simulink model "Marine_LocoMotive_UAV_est_git"  (R2018a)
settings: Solver=ode4  StartTime=0.0  StopTime=40  FixedStep=T  MaxStep=2*T  MinStep=T  RelTol=1e-4
values from neighbouring files (symbols this model uses):
  a_11 = 0.05*m_b    (= 0.625)    [Marine_LocoMotive_UAV_est_git_parameters.m]    (also in Marine_LocoMotive_UAV_medium_est_git_parameters.m = 1.6875; heave_dynamics_chart.m)
  a_33 = m_b    (= 12.5)    [Marine_LocoMotive_UAV_est_git_parameters.m]    (also in Marine_LocoMotive_UAV_medium_est_git_parameters.m = 33.75; heave_dynamics_chart.m)
  A_w = 1*3.3/2    (= 1.65)    [Marine_LocoMotive_UAV_est_git_parameters.m]    (also in Marine_LocoMotive_UAV_medium_est_git_parameters.m = 0.6)
  A_w2 = 1*1.2/2    (= 0.6)    [Marine_LocoMotive_UAV_est_git_parameters.m]    (also in Marine_LocoMotive_UAV_medium_est_git_parameters.m = 0.305)
  Ac = 0.0331    [Marine_LocoMotive_UAV_est_git_parameters.m]    (also in Marine_LocoMotive_UAV_medium_est_git_parameters.m = 0.422)
  alpha_bar = pi/4    (= 0.785398163397)    [Marine_LocoMotive_UAV_est_git_parameters.m]    (also in Marine_LocoMotive_UAV_medium_est_git_parameters.m; heave_dynamics_chart.m = pi/4*sign(V_bar(j)))
  Am = sysd.denominator{1}    [Marine_LocoMotive_UAV_est_git_parameters.m]    (also in Marine_LocoMotive_UAV_medium_est_git_parameters.m)
  Am1_LPF = sysd.denominator{1}    [Marine_LocoMotive_UAV_est_git_parameters.m]    (also in Marine_LocoMotive_UAV_medium_est_git_parameters.m)
  Am2_LPF = sysd.denominator{1}    [Marine_LocoMotive_UAV_est_git_parameters.m]    (also in Marine_LocoMotive_UAV_medium_est_git_parameters.m)
  Am_asw_LPF = sysd.denominator{1}    [Marine_LocoMotive_UAV_est_git_parameters.m]    (also in Marine_LocoMotive_UAV_medium_est_git_parameters.m)
  Am_coup_LPF = sysd.denominator{1}    [Marine_LocoMotive_UAV_est_git_parameters.m]    (also in Marine_LocoMotive_UAV_medium_est_git_parameters.m)
  Am_fast_coup_LPF = sysd.denominator{1}    [Marine_LocoMotive_UAV_est_git_parameters.m]    (also in Marine_LocoMotive_UAV_medium_est_git_parameters.m)
  Am_rdeL_LPF = sysd.denominator{1}    [Marine_LocoMotive_UAV_est_git_parameters.m]    (also in Marine_LocoMotive_UAV_medium_est_git_parameters.m)
  Am_reL_LPF = sysd.denominator{1}    [Marine_LocoMotive_UAV_est_git_parameters.m]    (also in Marine_LocoMotive_UAV_medium_est_git_parameters.m)
  Am_rref20_LPF = sysd.denominator{1}    [Marine_LocoMotive_UAV_est_git_parameters.m]    (also in Marine_LocoMotive_UAV_medium_est_git_parameters.m)
  Am_rref_LPF = sysd.denominator{1}    [Marine_LocoMotive_UAV_est_git_parameters.m]    (also in Marine_LocoMotive_UAV_medium_est_git_parameters.m)
  AmAlpha_LPF = sysd.denominator{1}    [Marine_LocoMotive_UAV_est_git_parameters.m]    (also in Marine_LocoMotive_UAV_medium_est_git_parameters.m)
  Amp_sf = 3    [Marine_LocoMotive_UAV_est_git_parameters.m]    (also in Marine_LocoMotive_UAV_medium_est_git_parameters.m)
  Amp_sf_rp = 0.05*m_u*g    (= 0.8829)    [Marine_LocoMotive_UAV_est_git_parameters.m]    (also in Marine_LocoMotive_UAV_medium_est_git_parameters.m = 9.56475)
  AmV_LPF = sysd.denominator{1}    [Marine_LocoMotive_UAV_est_git_parameters.m]    (also in Marine_LocoMotive_UAV_medium_est_git_parameters.m)
  AmZ_LPF = sysd.denominator{1}    [Marine_LocoMotive_UAV_est_git_parameters.m]    (also in Marine_LocoMotive_UAV_medium_est_git_parameters.m)
  b_11 = 0    [Marine_LocoMotive_UAV_est_git_parameters.m]    (also in Marine_LocoMotive_UAV_medium_est_git_parameters.m; heave_dynamics_chart.m)
  b_33 = 2*m_b*omega_h    (= 19.6349540849)    [Marine_LocoMotive_UAV_est_git_parameters.m]    (also in Marine_LocoMotive_UAV_medium_est_git_parameters.m = 84.8230016469; buoyancy_calc.m = 4.18879020479; heave_dynamics_chart.m = 2*m_b*omega_h)
  Bm = sysd.numerator{1}    [Marine_LocoMotive_UAV_est_git_parameters.m]    (also in Marine_LocoMotive_UAV_medium_est_git_parameters.m)
  Bm1_LPF = sysd.numerator{1}    [Marine_LocoMotive_UAV_est_git_parameters.m]    (also in Marine_LocoMotive_UAV_medium_est_git_parameters.m)
  Bm2_LPF = sysd.numerator{1}    [Marine_LocoMotive_UAV_est_git_parameters.m]    (also in Marine_LocoMotive_UAV_medium_est_git_parameters.m)
  Bm_asw_LPF = sysd.numerator{1}    [Marine_LocoMotive_UAV_est_git_parameters.m]    (also in Marine_LocoMotive_UAV_medium_est_git_parameters.m)
  Bm_coup_LPF = sysd.numerator{1}    [Marine_LocoMotive_UAV_est_git_parameters.m]    (also in Marine_LocoMotive_UAV_medium_est_git_parameters.m)
  Bm_fast_coup_LPF = sysd.numerator{1}    [Marine_LocoMotive_UAV_est_git_parameters.m]    (also in Marine_LocoMotive_UAV_medium_est_git_parameters.m)
  Bm_rdeL_LPF = sysd.numerator{1}    [Marine_LocoMotive_UAV_est_git_parameters.m]    (also in Marine_LocoMotive_UAV_medium_est_git_parameters.m)
  Bm_reL_LPF = sysd.numerator{1}    [Marine_LocoMotive_UAV_est_git_parameters.m]    (also in Marine_LocoMotive_UAV_medium_est_git_parameters.m)
  Bm_rref20_LPF = sysd.numerator{1}    [Marine_LocoMotive_UAV_est_git_parameters.m]    (also in Marine_LocoMotive_UAV_medium_est_git_parameters.m)
  Bm_rref_LPF = sysd.numerator{1}    [Marine_LocoMotive_UAV_est_git_parameters.m]    (also in Marine_LocoMotive_UAV_medium_est_git_parameters.m)
  BmAlpha_LPF = sysd.numerator{1}    [Marine_LocoMotive_UAV_est_git_parameters.m]    (also in Marine_LocoMotive_UAV_medium_est_git_parameters.m)
  BmV_LPF = sysd.numerator{1}    [Marine_LocoMotive_UAV_est_git_parameters.m]    (also in Marine_LocoMotive_UAV_medium_est_git_parameters.m)
  BmZ_LPF = sysd.numerator{1}    [Marine_LocoMotive_UAV_est_git_parameters.m]    (also in Marine_LocoMotive_UAV_medium_est_git_parameters.m)
  C_S = [5;9]*10^-3    [Marine_LocoMotive_UAV_est_git_parameters.m]    (also in Marine_LocoMotive_UAV_medium_est_git_parameters.m; heave_dynamics_chart.m = 0.075/(log10(Re)-2)^2)
  Cd_u = 0.2    [Marine_LocoMotive_UAV_est_git_parameters.m]    (also in Marine_LocoMotive_UAV_medium_est_git_parameters.m)
  D_x = b_11 + D_s(1)    [Marine_LocoMotive_UAV_est_git_parameters.m]    (also in Marine_LocoMotive_UAV_medium_est_git_parameters.m; heave_dynamics_chart.m = b_11 + D_s(i,j))
  D_z = b_33 + D_s(2)    [Marine_LocoMotive_UAV_est_git_parameters.m]    (also in Marine_LocoMotive_UAV_medium_est_git_parameters.m; heave_dynamics_chart.m)
  dc_M_p = 6.7    [Marine_LocoMotive_UAV_est_git_parameters.m]    (also in Marine_LocoMotive_UAV_medium_est_git_parameters.m)
  Delta_h = (A_im/A_b-0.5)*h_b    (= -0.0625)    [Marine_LocoMotive_UAV_est_git_parameters.m]    (also in Marine_LocoMotive_UAV_medium_est_git_parameters.m = -0.075; heave_dynamics_chart.m)
  eps_V = 0.1    [Marine_LocoMotive_UAV_est_git_parameters.m]    (also in Marine_LocoMotive_UAV_medium_est_git_parameters.m)
  epsilon_1 = 5    [Marine_LocoMotive_UAV_est_git_parameters.m]    (also in Marine_LocoMotive_UAV_medium_est_git_parameters.m)
  epsilon_e_u1 = 0.05    [Marine_LocoMotive_UAV_est_git_parameters.m]    (also in Marine_LocoMotive_UAV_medium_est_git_parameters.m)
  epsilon_w = 0    [Marine_LocoMotive_UAV_est_git_parameters.m]    (also in Marine_LocoMotive_UAV_medium_est_git_parameters.m)
  epsilon_w2 = pi    (= 3.14159265359)    [Marine_LocoMotive_UAV_est_git_parameters.m]    (also in Marine_LocoMotive_UAV_medium_est_git_parameters.m)
  g = 9.81    [Marine_LocoMotive_UAV_est_git_parameters.m]    (also in Marine_LocoMotive_UAV_medium_est_git_parameters.m; heave_dynamics_chart.m)
  gamma_d_p = (2*0.3/0.03*2*0.2*12/4)/10    (= 2.4)    [Marine_LocoMotive_UAV_est_git_parameters.m]    (also in Marine_LocoMotive_UAV_medium_est_git_parameters.m)
  H = 10    [Marine_LocoMotive_UAV_est_git_parameters.m]    (also in Marine_LocoMotive_UAV_medium_est_git_parameters.m)
  h_b = 0.25    [Marine_LocoMotive_UAV_est_git_parameters.m]    (also in Marine_LocoMotive_UAV_medium_est_git_parameters.m = 0.3; buoyancy_calc.m = 0.15; heave_dynamics_chart.m)
  J_b = m_b*h_b*l_b/12    (= 0.208333333333)    [Marine_LocoMotive_UAV_est_git_parameters.m]    (also in Marine_LocoMotive_UAV_medium_est_git_parameters.m = 1.265625; heave_dynamics_chart.m)
  J_u = 0.03    [Marine_LocoMotive_UAV_est_git_parameters.m]    (also in Marine_LocoMotive_UAV_medium_est_git_parameters.m = 1.51708333333)
  K = 40    [Marine_LocoMotive_UAV_est_git_parameters.m]    (also in Marine_LocoMotive_UAV_medium_est_git_parameters.m = 83.3333333333)
  k3 = 24    [Marine_LocoMotive_UAV_est_git_parameters.m]    (also in Marine_LocoMotive_UAV_medium_est_git_parameters.m)
  k4 = 0.8    [Marine_LocoMotive_UAV_est_git_parameters.m]    (also in Marine_LocoMotive_UAV_medium_est_git_parameters.m)
  k_w = omega_w^2/g    (= 0.0628797426165)    [Marine_LocoMotive_UAV_est_git_parameters.m]    (also in Marine_LocoMotive_UAV_medium_est_git_parameters.m = 0.160972141098; heave_dynamics_chart.m = omega_w^2/g)
  k_w2 = omega_w2^2/g    (= 0.160972141098)    [Marine_LocoMotive_UAV_est_git_parameters.m]    (also in Marine_LocoMotive_UAV_medium_est_git_parameters.m = 0.251518970466)
  kd_a = 5.6    [Marine_LocoMotive_UAV_est_git_parameters.m]    (also in Marine_LocoMotive_UAV_medium_est_git_parameters.m)
  kd_r = 19.5    [Marine_LocoMotive_UAV_est_git_parameters.m]    (also in Marine_LocoMotive_UAV_medium_est_git_parameters.m)
  kd_t = 10    [Marine_LocoMotive_UAV_est_git_parameters.m]    (also in Marine_LocoMotive_UAV_medium_est_git_parameters.m = 25)
  kd_x = 5    [Marine_LocoMotive_UAV_est_git_parameters.m]    (also in Marine_LocoMotive_UAV_medium_est_git_parameters.m)
  kd_z = 2    [Marine_LocoMotive_UAV_est_git_parameters.m]    (also in Marine_LocoMotive_UAV_medium_est_git_parameters.m)
  ki_a = 1.6    [Marine_LocoMotive_UAV_est_git_parameters.m]    (also in Marine_LocoMotive_UAV_medium_est_git_parameters.m)
  ki_r = 9    [Marine_LocoMotive_UAV_est_git_parameters.m]    (also in Marine_LocoMotive_UAV_medium_est_git_parameters.m)
  ki_T = 12    [Marine_LocoMotive_UAV_est_git_parameters.m]    (also in Marine_LocoMotive_UAV_medium_est_git_parameters.m)
  ki_x = 1.2    [Marine_LocoMotive_UAV_est_git_parameters.m]    (also in Marine_LocoMotive_UAV_medium_est_git_parameters.m)
  ki_z = 1    [Marine_LocoMotive_UAV_est_git_parameters.m]    (also in Marine_LocoMotive_UAV_medium_est_git_parameters.m)
  kp_a = 9.6    [Marine_LocoMotive_UAV_est_git_parameters.m]    (also in Marine_LocoMotive_UAV_medium_est_git_parameters.m)
  kp_r = 45    [Marine_LocoMotive_UAV_est_git_parameters.m]    (also in Marine_LocoMotive_UAV_medium_est_git_parameters.m)
  kp_t = 20    [Marine_LocoMotive_UAV_est_git_parameters.m]    (also in Marine_LocoMotive_UAV_medium_est_git_parameters.m = 50)
  kp_T = 25    [Marine_LocoMotive_UAV_est_git_parameters.m]    (also in Marine_LocoMotive_UAV_medium_est_git_parameters.m)
  kp_x = 7    [Marine_LocoMotive_UAV_est_git_parameters.m]    (also in Marine_LocoMotive_UAV_medium_est_git_parameters.m)
  kp_z = 3    [Marine_LocoMotive_UAV_est_git_parameters.m]    (also in Marine_LocoMotive_UAV_medium_est_git_parameters.m)
  L = 0.2    [Marine_LocoMotive_UAV_est_git_parameters.m]    (also in Marine_LocoMotive_UAV_medium_est_git_parameters.m = 0.8)
  l_b = 0.8    [Marine_LocoMotive_UAV_est_git_parameters.m]    (also in Marine_LocoMotive_UAV_medium_est_git_parameters.m = 1.5; buoyancy_calc.m = 0.5; heave_dynamics_chart.m)
  Lc_0 = 7    [Marine_LocoMotive_UAV_est_git_parameters.m]    (also in Marine_LocoMotive_UAV_medium_est_git_parameters.m = 20)
  LIMIT_CMD_PITCH = 45*pi/180    (= 0.785398163397)    [Marine_LocoMotive_UAV_est_git_parameters.m]    (also in Marine_LocoMotive_UAV_medium_est_git_parameters.m)
  LIMIT_uCMD_HEIGHT = 0.9*n_motors*K    (= 144)    [Marine_LocoMotive_UAV_est_git_parameters.m]    (also in Marine_LocoMotive_UAV_medium_est_git_parameters.m = 450)
  m_b = rho_w*Vol_b/4    (= 12.5)    [Marine_LocoMotive_UAV_est_git_parameters.m]    (also in Marine_LocoMotive_UAV_medium_est_git_parameters.m = 33.75; buoyancy_calc.m = 5; heave_dynamics_chart.m)
  m_u = 1.8    [Marine_LocoMotive_UAV_est_git_parameters.m]    (also in Marine_LocoMotive_UAV_medium_est_git_parameters.m = 19.5)
  min_sf = 5    [Marine_LocoMotive_UAV_est_git_parameters.m]    (also in Marine_LocoMotive_UAV_medium_est_git_parameters.m)
  min_sf_rp = 0.35*m_u*g    (= 6.1803)    [Marine_LocoMotive_UAV_est_git_parameters.m]    (also in Marine_LocoMotive_UAV_medium_est_git_parameters.m = 66.95325)
  n_motors = 4    [Marine_LocoMotive_UAV_est_git_parameters.m]    (also in Marine_LocoMotive_UAV_medium_est_git_parameters.m = 6)
  nu_w = 1.787*10^-6    (= 1.787e-06)    [Marine_LocoMotive_UAV_est_git_parameters.m]    (also in Marine_LocoMotive_UAV_medium_est_git_parameters.m; buoyancy_calc.m; heave_dynamics_chart.m)
  omega_w = 2*pi/T_w    (= 0.785398163397)    [Marine_LocoMotive_UAV_est_git_parameters.m]    (also in Marine_LocoMotive_UAV_medium_est_git_parameters.m = 1.25663706144; heave_dynamics_chart.m = 2*pi/T_i)
  omega_w2 = 2*pi/T_w2    (= 1.25663706144)    [Marine_LocoMotive_UAV_est_git_parameters.m]    (also in Marine_LocoMotive_UAV_medium_est_git_parameters.m = 1.57079632679)
  r_0 = sqrt( (X0_b(1) - X0_u(1))^2 +(X0_b(2) - X0_u(2))^2 )    [Marine_LocoMotive_UAV_est_git_parameters.m]    (also in Marine_LocoMotive_UAV_medium_est_git_parameters.m)
  R_b = 0.1    [buoyancy_calc.m]
  r_bar = Lc_0-0.3    (= 6.7)    [Marine_LocoMotive_UAV_est_git_parameters.m]    (also in Marine_LocoMotive_UAV_medium_est_git_parameters.m = 19.7)
  r_min = (zu_bar-H)-0.2    [Marine_LocoMotive_UAV_est_git_parameters.m]    (also in Marine_LocoMotive_UAV_medium_est_git_parameters.m)
  rho_a = 1.225    [Marine_LocoMotive_UAV_est_git_parameters.m]    (also in Marine_LocoMotive_UAV_medium_est_git_parameters.m)
  rho_w = 1000    [Marine_LocoMotive_UAV_est_git_parameters.m]    (also in Marine_LocoMotive_UAV_medium_est_git_parameters.m; buoyancy_calc.m; heave_dynamics_chart.m)
  T = 1/500    (= 0.002)    [Marine_LocoMotive_UAV_est_git_parameters.m]    (also in Marine_LocoMotive_UAV_medium_est_git_parameters.m)
  T_init = 10    [Marine_LocoMotive_UAV_est_git_parameters.m]    (also in Marine_LocoMotive_UAV_medium_est_git_parameters.m)
  Theta0 = 0    [Marine_LocoMotive_UAV_est_git_parameters.m]    (also in Marine_LocoMotive_UAV_medium_est_git_parameters.m)
  torque_corr = 2*cosd(60)+1    [Marine_LocoMotive_UAV_est_git_parameters.m]    (also in Marine_LocoMotive_UAV_medium_est_git_parameters.m)
  u_s = w_dir*A_w^2*omega_w*k_w*exp(2*k_w*(-Delta_h/2))    [Marine_LocoMotive_UAV_est_git_parameters.m]    (also in Marine_LocoMotive_UAV_medium_est_git_parameters.m)
  u_s2 = w_dir2*A_w2^2*omega_w2*k_w2*exp(2*k_w2*(-Delta_h/2))    [Marine_LocoMotive_UAV_est_git_parameters.m]    (also in Marine_LocoMotive_UAV_medium_est_git_parameters.m)
  u_t = -1*0.5*1    (= -0.5)    [Marine_LocoMotive_UAV_est_git_parameters.m]    (also in Marine_LocoMotive_UAV_medium_est_git_parameters.m)
  u_w = 0*0.2    (= 0)    [Marine_LocoMotive_UAV_est_git_parameters.m]    (also in Marine_LocoMotive_UAV_medium_est_git_parameters.m)
  V0_b = [u_t+u_w+u_s+v_x_w, v_z_w].*[1 1]    [Marine_LocoMotive_UAV_est_git_parameters.m]    (also in Marine_LocoMotive_UAV_medium_est_git_parameters.m = [u_t+u_w+u_s+v_x_w, v_z_w])
  V0_u = V0_b    [Marine_LocoMotive_UAV_est_git_parameters.m]    (also in Marine_LocoMotive_UAV_medium_est_git_parameters.m = [0 0])
  V_bar = 4    [Marine_LocoMotive_UAV_est_git_parameters.m]    (also in Marine_LocoMotive_UAV_medium_est_git_parameters.m; heave_dynamics_chart.m = [-20:0.1:20]')
  Vol_b = A_b*l_b    (= 0.05)    [Marine_LocoMotive_UAV_est_git_parameters.m]    (also in Marine_LocoMotive_UAV_medium_est_git_parameters.m = 0.135; heave_dynamics_chart.m)
  w_dir = 1    [Marine_LocoMotive_UAV_est_git_parameters.m]    (also in Marine_LocoMotive_UAV_medium_est_git_parameters.m; heave_dynamics_chart.m)
  w_dir2 = 1    [Marine_LocoMotive_UAV_est_git_parameters.m]    (also in Marine_LocoMotive_UAV_medium_est_git_parameters.m)
  X0_b = [0,H-Delta_h]    [Marine_LocoMotive_UAV_est_git_parameters.m]    (also in Marine_LocoMotive_UAV_medium_est_git_parameters.m)
  X0_u = X0_b + [3/7 3/7]*Lc_0    [Marine_LocoMotive_UAV_est_git_parameters.m]    (also in Marine_LocoMotive_UAV_medium_est_git_parameters.m)
  zu_bar = X0_b(2) + Lc_0*sin(alpha_bar_0)    [Marine_LocoMotive_UAV_est_git_parameters.m]    (also in Marine_LocoMotive_UAV_medium_est_git_parameters.m)
undefined symbols (not defined in the file or in its folder): Am_HPF, Am_LPF, Am_LPF2, an1, an1_v, an2, an3, Bm_HPF, Bm_LPF, Bm_LPF2, bn1, bn1_v, bn2, bn3, DiscIntNeverNeededParam, F, Light, magnitude, MIL, OMEGA_FILTER_OUTER, Tc, Tg, Tn, Ts, Tsc, Tz, X_GPS_offset
libraries: simulink x55, simulink_extras x9, aerolibwind2 x2
(part 6 of 9)

== system Marine_LocoMotive_UAV_est_git/Sensors and Filters/Sensors/Gyro (500Hz) ==
  q : Inport
  Degrees to Radians2 : simulink_extras/Transformations/Degrees to Radians
  From File1 : FromFile  FileName=gyro_q_noise.mat  SampleTime=Tz
  Manual Switch1 : ManualSwitch
  Manual Switch5 : ManualSwitch  CurrentSetting=0
  Product1 : Product  SaturateOnIntegerOverflow=on  RndMeth=Zero  InputSameDT=on  OutDataTypeStr=Inherit: Same as first input
  Slider Gain1 : simulink/Math Operations/Slider Gain  gain=1  low=0  high=2
  Sum2 : Sum  Inputs=+++  SaturateOnIntegerOverflow=on  InputSameDT=on  OutDataTypeStr=Inherit: Same as first input
  Variable Integer Delay3 : Delay  DelayLength=0
  bias1 : Constant  Value=-1  VectorParams1D=off
  bias2 : Constant  Value=0  VectorParams1D=off
  bias5 : Constant  Value=0.9  VectorParams1D=off
  bias9 : Constant  VectorParams1D=off
  " q" : Outport
  wires:
  bias9/1 -> Manual Switch5/2
  bias5/1 -> Manual Switch5/1
  Manual Switch1/1 -> Degrees to Radians2/1
  bias2/1 -> Manual Switch1/2
  bias1/1 -> Manual Switch1/1
  Degrees to Radians2/1 -> Sum2/2
  Manual Switch5/1 -> Product1/1
  Sum2/1 -> Product1/2
  From File1/1 -> Slider Gain1/1
  Product1/1 -> Variable Integer Delay3/1
  Variable Integer Delay3/1 -> " q"/1
  Slider Gain1/1 -> Sum2/1
  q/1 -> Sum2/3

== system Marine_LocoMotive_UAV_est_git/Sensors and Filters/Sensors/rotation matrix R ==
  angle (rad) : Inport
  Gain : Gain  Gain=-1
  Signal Specification1 : SignalSpecification  Dimensions=2
  Signal Specification2 : SignalSpecification  Dimensions=2
  Trigonometric Function1 : Trigonometry  Operator=sincos
  Vector Concatenate1 : Concatenate  Mode=Multidimensional array  ConcatenateDimension=2
  Vector Concatenate2 : Concatenate
  Vector Concatenate3 : Concatenate
  R : Outport
  wires:
  Signal Specification2/1 -> Vector Concatenate1/2
  Signal Specification1/1 -> Vector Concatenate1/1
  Vector Concatenate1/1 -> R/1
  Vector Concatenate2/1 -> Signal Specification1/1
  Vector Concatenate3/1 -> Signal Specification2/1
  angle (rad)/1 -> Trigonometric Function1/1
  Trigonometric Function1/2 -> Vector Concatenate3/2, Vector Concatenate2/1
  Trigonometric Function1/1 -> Vector Concatenate2/2, Gain/1
  Gain/1 -> Vector Concatenate3/1

== system Marine_LocoMotive_UAV_est_git/Sensors and Filters/quadrotor position from relative buoy-UAV position/rotation matrix R  ==
  angle (rad) : Inport
  Gain2 : Gain  Gain=-1
  Signal Specification1 : SignalSpecification  Dimensions=2
  Signal Specification2 : SignalSpecification  Dimensions=2
  Trigonometric Function1 : Trigonometry  Operator=sincos
  Vector Concatenate1 : Concatenate  Mode=Multidimensional array  ConcatenateDimension=2
  Vector Concatenate2 : Concatenate
  Vector Concatenate3 : Concatenate
  R : Outport
  wires:
  Signal Specification2/1 -> Vector Concatenate1/2
  Signal Specification1/1 -> Vector Concatenate1/1
  Vector Concatenate2/1 -> Signal Specification1/1
  Vector Concatenate3/1 -> Signal Specification2/1
  angle (rad)/1 -> Trigonometric Function1/1
  Trigonometric Function1/2 -> Vector Concatenate2/1, Vector Concatenate3/2
  Vector Concatenate1/1 -> R/1
  Trigonometric Function1/1 -> Vector Concatenate2/2, Gain2/1
  Gain2/1 -> Vector Concatenate3/1

== system Marine_LocoMotive_UAV_est_git/UAV controller/Coupling/Coupling ==
  note: atan({U1.sin_psi-U2.cos_psi}/U3)
      |
      | asin{(U2.sin_psi+U1.cos_psi)/u1}
  U1 : Inport
  U3 : Inport  Port=2
  Add5 : Sum  Inputs=2
  Divide1 : Product  Inputs=*/
  Gain : Gain  Gain=m_u
  Product4 : Product
  Product5 : Product
  Saturation : Saturate  UpperLimit=LIMIT_uCMD_HEIGHT  LowerLimit=m_u*g*0.5
  Scope : Scope
  Scope1 : Scope
  Sqrt1 : Sqrt  SaturateOnIntegerOverflow=on
  Trigonometric Function2 : Trigonometry  Operator=atan
  u1 (N) : Outport
  phi_d (rad) : Outport  Port=2
  wires:
  U1/1 -> Divide1/1, Product4/2, Product4/1
  Divide1/1 -> Trigonometric Function2/1
  Trigonometric Function2/1 -> phi_d (rad)/1
  Product4/1 -> Add5/1, Scope/1
  Sqrt1/1 -> Gain/1
  Product5/1 -> Scope1/1, Add5/2
  Add5/1 -> Sqrt1/1
  U3/1 -> Divide1/2, Product5/1, Product5/2
  Saturation/1 -> u1 (N)/1
  Gain/1 -> Saturation/1

== system Marine_LocoMotive_UAV_est_git/UAV controller/Coupling/sat ==
  u : Inport
  Fcn1 : Fcn  Expr=LIMIT_CMD_PITCH*tanh(u(1)/LIMIT_CMD_PITCH)
  Manual Switch : ManualSwitch
  Saturation1 : Saturate  UpperLimit=LIMIT_CMD_PITCH  LowerLimit=-LIMIT_CMD_PITCH
  sat(u) : Outport
  wires:
  u/1 -> Fcn1/1, Saturation1/1
  Manual Switch/1 -> sat(u)/1
  Saturation1/1 -> Manual Switch/2
  Fcn1/1 -> Manual Switch/1

== system Marine_LocoMotive_UAV_est_git/UAV controller/Coupling /Subsystem2 ==
  u_a : Inport
  alpha : Inport  Port=2
  theta_q : Inport  Port=3
  u_T : Inport  Port=4
  alpha 1 : Inport  Port=5
  Add : Sum
  Add1 : Sum  Inputs=+-
  Compare To Constant : simulink/Logic and Bit Operations/Compare To Constant  relop=>=  const=pi/2  OutDataTypeStr=boolean
  Compare To Constant1 : simulink/Logic and Bit Operations/Compare To Constant  relop=<=  const=pi/2  OutDataTypeStr=boolean
  Delay : Delay  DelayLength=1
  Logical Operator : Logic  AllPortsSameDT=off  OutDataTypeStr=boolean
  MATLAB Function : MATLAB Function  TreatAsAtomicUnit=on
  MinMax : MinMax  Function=max  Inputs=2
  Product{1..4} (4 alike) : Product
  Relational Operator : RelationalOperator  Operator=<=  OutDataTypeStr=boolean  RndMeth=Simplest
  Saturation : Saturate  UpperLimit=inf  LowerLimit=0
  Sqrt1 : Sqrt  SaturateOnIntegerOverflow=on
  Switch : Switch  Criteria=u2 > Threshold  Threshold=pi/2
  Trigonometric Function : Trigonometry  Operator=cos
  Trigonometric Function1 : Trigonometry  Operator=cos
  "alpha " : InportShadow  Port=2
  smooth switch : Subsystem
  u_1_min : Constant  Value=m_u*g*0.5
  u_1_min1 : Constant  Value=m_u*g
  u_1_min2 : Constant  Value=m_u*g
  u_a_out : Outport
  wires:
  Relational Operator/1 -> Logical Operator/2
  Product3/1 -> Relational Operator/2
  u_1_min2/1 -> Product3/1
  Trigonometric Function1/1 -> Product3/2
  alpha 1/1 -> Trigonometric Function1/1
  Product1/1 -> MinMax/1
  "alpha "/1 -> Trigonometric Function/1
  Trigonometric Function/1 -> Product1/2
  u_1_min1/1 -> Product1/1
  Add1/1 -> Saturation/1
  u_a/1 -> smooth switch/1(u 1), Relational Operator/1, MinMax/2
  Add/1 -> Compare To Constant/1, Compare To Constant1/1
  Product2/1 -> Add1/1
  u_1_min/1 -> Product2/2, Product2/1
  smooth switch/1(y) -> u_a_out/1
  Compare To Constant1/1 -> Switch/3
  Sqrt1/1 -> smooth switch/2(u 2)  "u_a_min"
  theta_q/1 -> Add/2
  u_T/1 -> Product4/1, Product4/2
  Logical Operator/1 -> smooth switch/3(switch)
  Product4/1 -> Add1/2
  alpha/1 -> Delay/1, Add/1
  Saturation/1 -> Sqrt1/1
  Delay/1 -> Switch/2
  Switch/1 -> Logical Operator/1
  Compare To Constant/1 -> Switch/1

== system Marine_LocoMotive_UAV_est_git/UAV controller/Coupling /Subsystem3 ==
  u_a : Inport
  alpha : Inport  Port=2
  theta_q : Inport  Port=3
  u_T : Inport  Port=4
  Add : Sum
  Add1 : Sum  Inputs=+-
  Compare To Constant : simulink/Logic and Bit Operations/Compare To Constant  relop=<=  const=pi  OutDataTypeStr=boolean
  Compare To Zero : simulink/Logic and Bit Operations/Compare To Zero  relop=>=  OutDataTypeStr=boolean
  Compare To Zero1 : simulink/Logic and Bit Operations/Compare To Zero  relop=<=  OutDataTypeStr=boolean
  Delay : Delay  DelayLength=1
  Logical Operator : Logic  AllPortsSameDT=off  OutDataTypeStr=boolean
  MATLAB Function : MATLAB Function  TreatAsAtomicUnit=on
  Product2 : Product
  Product4 : Product
  Saturation : Saturate  UpperLimit=inf  LowerLimit=0
  Scope5 : Scope
  Sqrt1 : Sqrt  SaturateOnIntegerOverflow=on
  Switch : Switch  Criteria=u2 > Threshold  Threshold=pi/2
  Vector Concatenate : Concatenate  NumInputs=3
  g : Constant  Value=g
  m_u : Constant  Value=m_u
  smooth switch : Subsystem
  u_1_min : Constant  Value=m_u*g*0.5
  u_T_out : Outport
  wires:
  m_u/1 -> MATLAB Function/4(m_q)
  g/1 -> MATLAB Function/5(g)
  Vector Concatenate/1 -> Scope5/1
  Compare To Constant/1 -> Switch/1
  Switch/1 -> Logical Operator/1
  Delay/1 -> Switch/2
  Saturation/1 -> Sqrt1/1
  u_T/1 -> Compare To Zero1/1, smooth switch/1(u 1), Vector Concatenate/1
  alpha/1 -> Add/1, Delay/1
  Product4/1 -> Add1/2
  Logical Operator/1 -> smooth switch/3(switch)
  u_a/1 -> Product4/2, Product4/1
  theta_q/1 -> Add/2
  Sqrt1/1 -> smooth switch/2(u 2), Vector Concatenate/2  "u_T_min"
  Compare To Zero/1 -> Switch/3
  smooth switch/1(y) -> u_T_out/1, Vector Concatenate/3
  u_1_min/1 -> Product2/1, Product2/2
  Product2/1 -> Add1/1
  Add/1 -> Compare To Zero/1, Compare To Constant/1
  Compare To Zero1/1 -> Logical Operator/2
  Add1/1 -> Saturation/1

== system Marine_LocoMotive_UAV_est_git/UAV controller/Coupling /sat  ==
  u : Inport
  Fcn1 : Fcn  Expr=LIMIT_CMD_PITCH*tanh(u(1)/LIMIT_CMD_PITCH)
  Manual Switch : ManualSwitch
  Saturation1 : Saturate  UpperLimit=LIMIT_CMD_PITCH  LowerLimit=-LIMIT_CMD_PITCH
  sat(u) : Outport
  wires:
  u/1 -> Fcn1/1, Saturation1/1
  Manual Switch/1 -> sat(u)/1
  Saturation1/1 -> Manual Switch/2
  Fcn1/1 -> Manual Switch/1

== system Marine_LocoMotive_UAV_est_git/UAV controller/Coupling /u_T switch ==
  alpha : Inport
  theta_q : Inport  Port=2
  u_T : Inport  Port=3
  MATLAB Function : MATLAB Function  TreatAsAtomicUnit=on
  Manual Switch : ManualSwitch
  Scope5 : Scope
  Vector Concatenate : Concatenate  NumInputs=3
  g : Constant  Value=g
  m_u : Constant  Value=m_u
  smooth switch : Subsystem
  u_T_out : Outport
  wires:
  smooth switch/1(y) -> Manual Switch/2, Vector Concatenate/3
  alpha/1 -> MATLAB Function/2(alpha)
  Vector Concatenate/1 -> Scope5/1
  g/1 -> MATLAB Function/5(g)
  m_u/1 -> MATLAB Function/4(m_q)
  u_T/1 -> Manual Switch/1, Vector Concatenate/1, smooth switch/1(u 1), MATLAB Function/1(u_T)
  theta_q/1 -> MATLAB Function/3(theta_u)
  MATLAB Function/1(u_T_out) -> Vector Concatenate/2, smooth switch/2(u 2)
  MATLAB Function/2(c) -> smooth switch/3(switch)
  Manual Switch/1 -> u_T_out/1

== system Marine_LocoMotive_UAV_est_git/UAV controller/Coupling /u_a switch ==
  u_a : Inport
  alpha : Inport  Port=2
  theta_q : Inport  Port=3
  MATLAB Function : MATLAB Function  TreatAsAtomicUnit=on
  Manual Switch : ManualSwitch
  Scope1 : Scope
  Scope5 : Scope
  Vector Concatenate : Concatenate  NumInputs=3
  g : Constant  Value=g
  m_u : Constant  Value=m_u
  smooth switch : Subsystem
  u_a_out : Outport
  wires:
  MATLAB Function/2(c) -> Scope1/1, smooth switch/3(switch)
  g/1 -> MATLAB Function/5(g)
  alpha/1 -> MATLAB Function/2(alpha)
  theta_q/1 -> MATLAB Function/3(theta_u)
  m_u/1 -> MATLAB Function/4(m_q)
  u_a/1 -> Vector Concatenate/1, Manual Switch/1, smooth switch/1(u 1), MATLAB Function/1(u_a)
  MATLAB Function/1(u_a_out) -> Vector Concatenate/2, smooth switch/2(u 2)
  smooth switch/1(y) -> Vector Concatenate/3, Manual Switch/2
  Vector Concatenate/1 -> Scope5/1
  Manual Switch/1 -> u_a_out/1

== system Marine_LocoMotive_UAV_est_git/UAV controller/switch controllers/Smooth channel switching ==
  c1 : Inport
  switch : Inport  Port=2
  c2 : Inport  Port=3
  C1 transition : Subsystem
  C2 transition : Subsystem
  Delay : Delay  DelayLength=1
  Delay1 : Delay  DelayLength=1
  Logical Operator : Logic  Operator=NOT  AllPortsSameDT=off  OutDataTypeStr=boolean
  Mux3 : Mux  Inputs=3
  "c1,c2, u_out" : Scope
  c2 out if switch is 1 : Switch  Criteria=u2 > Threshold
  u_out : Outport
  wires:
  C2 transition/1(C2_trans) -> [c2_trans]  "C2 s"
  Logical Operator/1 -> C1 transition/2(switch)
  Delay1/1 -> C1 transition/3(C2_0)
  Delay/1 -> C2 transition/3(C1_0)
  Mux3/1 -> "c1,c2, u_out"/1
  switch/1 -> C2 transition/2(switch), Logical Operator/1, c2 out if switch is 1/2
  c2/1 -> C2 transition/1(C2), Mux3/2
  c2 out if switch is 1/1 -> u_out/1, Mux3/3  "out"
  c1/1 -> C1 transition/1(C1), Mux3/1
  C1 transition/1(C1_trans) -> [c1_trans]
  [c2_trans] -> Delay1/1
  [c1_trans] -> Delay/1
  [c1_trans] -> c2 out if switch is 1/3
  [c2_trans] -> c2 out if switch is 1/1

== system Marine_LocoMotive_UAV_est_git/UAV controller/switch controllers/smooth switch ==
  u 1 : Inport
  u 2 : Inport  Port=2
  switch : Inport  Port=3
  Constant : Constant
  Data Type Conversion : DataTypeConversion
  Low Pass Filter2 : DiscreteTransferFcn  Numerator=Bm_coup_LPF  Denominator=Am_coup_LPF
  Product : Product
  Product1 : Product
  Step1 : Step  SampleTime=0
  Subtract : Sum  Inputs=+-
  Sum : Sum  Inputs=|++
  "switch " : Scope
  y : Outport
  wires:
  Product/1 -> Sum/2
  Product1/1 -> Sum/1
  Low Pass Filter2/1 -> "switch "/1, Product/1, Subtract/2
  Data Type Conversion/1 -> Low Pass Filter2/1
  u 1/1 -> Product1/1
  u 2/1 -> Product/2
  switch/1 -> Data Type Conversion/1
  Sum/1 -> y/1
  Constant/1 -> Subtract/1
  Subtract/1 -> Product1/2

== system Marine_LocoMotive_UAV_est_git/UAV controller/u_a_Lyapunov/Subsystem ==
  In1 : Inport
  smothing : DiscreteTransferFcn  Numerator=Bm_coup_LPF  Denominator=Am_coup_LPF
  Out1 : Outport
  wires:
  smothing/1 -> Out1/1
  In1/1 -> smothing/1

== system Marine_LocoMotive_UAV_est_git/UAV controller/u_a_Lyapunov/Subsystem1 ==
  alpha_ref_ddot : Inport
  reset : Inport  Port=2
  Delay3 : Delay  Commented=on  DelayLength=1  InitialCondition=0
  Enabled Subsystem1 : Subsystem  Commented=on  TreatAsAtomicUnit=on
  Low Pass Filter5 : DiscreteTransferFcn  Numerator=Bm_rdeL_LPF  Denominator=Am_rdeL_LPF
  Switch : Switch  Commented=on  Criteria=u2 > Threshold
  alpha 0 : Subsystem  Commented=on  TreatAsAtomicUnit=on
  cond1 : Subsystem  Commented=on
  Out1 : Outport
  wires:
  reset/1 -> Delay3/1
  cond1/1(key) -> alpha 0/Trigger, Enabled Subsystem1/Enable, Switch/2
  Low Pass Filter5/1 -> Out1/1
  Delay3/1 -> Enabled Subsystem1/2(reset)
  alpha 0/1(Xu_init) -> Enabled Subsystem1/3(u0)
  Enabled Subsystem1/1(y) -> Switch/1
  alpha_ref_ddot/1 -> Low Pass Filter5/1, Switch/3, Enabled Subsystem1/1(u), alpha 0/1(X)

== system Marine_LocoMotive_UAV_est_git/UAV controller/u_a_Lyapunov/smooth lower bound ==
  u : Inport
  Manual Switch : ManualSwitch  CurrentSetting=0
  Mux3 : Mux  Inputs=2
  Saturation8 : Saturate  UpperLimit=0  LowerLimit=-25*m_u
  apply for lower bound only : Switch  Criteria=u2 > Threshold  Threshold=Amp_sf+0
  sat : Scope
  saturation function : Fcn  Expr=Amp_sf*tanh((u(1)-(Amp_sf+0))/(Amp_sf)) + (Amp_sf+0)
  sat(u) : Outport
  wires:
  Manual Switch/1 -> sat(u)/1
  Saturation8/1 -> Manual Switch/2
  u/1 -> saturation function/1, apply for lower bound only/2, Saturation8/1, Mux3/1, apply for lower bound only/1
  saturation function/1 -> apply for lower bound only/3, Mux3/2
  Mux3/1 -> sat/1
  apply for lower bound only/1 -> Manual Switch/1

== system Marine_LocoMotive_UAV_est_git/UAV controller/u_a_Lyapunov/smooth lower bound1 ==
  u : Inport
  Manual Switch : ManualSwitch  CurrentSetting=0
  Mux3 : Mux  Inputs=2
  Saturation7 : Saturate  UpperLimit=25*m_u  LowerLimit=0
  apply for lower bound only : Switch  Criteria=u2 > Threshold  Threshold=Amp_sf+min_sf
  sat : Scope
  saturation function : Fcn  Expr=Amp_sf*tanh((u(1)+(Amp_sf+min_sf))/(Amp_sf)) + (Amp_sf+min_sf)
  sat(u) : Outport
  wires:
  apply for lower bound only/1 -> Manual Switch/1
  Mux3/1 -> sat/1
  saturation function/1 -> Mux3/2, apply for lower bound only/3
  u/1 -> Saturation7/1, apply for lower bound only/1, Mux3/1, apply for lower bound only/2, saturation function/1
  Saturation7/1 -> Manual Switch/2
  Manual Switch/1 -> sat(u)/1

== system Marine_LocoMotive_UAV_est_git/UAV controller/u_r_V_Lyapunov buoy velocity/Smooth channel switching1 ==
  c1 : Inport
  switch : Inport  Port=2
  c2 : Inport  Port=3
  C1 transition : Subsystem
  C2 transition : Subsystem
  Delay : Delay  DelayLength=1
  Delay1 : Delay  DelayLength=1
  Logical Operator : Logic  Operator=NOT  AllPortsSameDT=off  OutDataTypeStr=boolean
  Mux3 : Mux  Inputs=3
  "c1,c2, u_out" : Scope
  c2 out if switch is 1 : Switch  Criteria=u2 > Threshold
  u_out : Outport
  wires:
  [c2_trans] -> c2 out if switch is 1/1
  [c1_trans] -> c2 out if switch is 1/3
  [c1_trans] -> Delay/1
  [c2_trans] -> Delay1/1
  C1 transition/1(C1_trans) -> [c1_trans]
  c1/1 -> Mux3/1, C1 transition/1(C1)
  c2 out if switch is 1/1 -> Mux3/3, u_out/1  "out"
  c2/1 -> Mux3/2, C2 transition/1(C2)
  switch/1 -> c2 out if switch is 1/2, Logical Operator/1, C2 transition/2(switch)
  Mux3/1 -> "c1,c2, u_out"/1
  Delay/1 -> C2 transition/3(C1_0)
  Delay1/1 -> C1 transition/3(C2_0)
  Logical Operator/1 -> C1 transition/2(switch)
  C2 transition/1(C2_trans) -> [c2_trans]  "C2 s"

== system Marine_LocoMotive_UAV_est_git/UAV controller/u_r_V_Lyapunov buoy velocity/Subsystem ==
  In1 : Inport
  smothing : DiscreteTransferFcn  Numerator=Bm_coup_LPF  Denominator=Am_coup_LPF
  Out1 : Outport
  wires:
  smothing/1 -> Out1/1
  In1/1 -> smothing/1

== system Marine_LocoMotive_UAV_est_git/UAV controller/u_r_V_Lyapunov buoy velocity/Subsystem1 ==
  In1 : Inport
  smothing : DiscreteTransferFcn  Numerator=Bm_coup_LPF  Denominator=Am_coup_LPF
  Out1 : Outport
  wires:
  In1/1 -> smothing/1
  smothing/1 -> Out1/1

== system Marine_LocoMotive_UAV_est_git/UAV controller/u_r_V_Lyapunov buoy velocity/smooth lower bound ==
  u : Inport
  Manual Switch : ManualSwitch
  Mux3 : Mux  Inputs=2
  Saturation1 : Saturate  UpperLimit=inf  LowerLimit=min_sf
  apply for lower bound only : Switch  Criteria=u2 > Threshold  Threshold=Amp_sf+min_sf
  sat : Scope
  saturation function : Fcn  Expr=Amp_sf*tanh((u(1)-(Amp_sf+min_sf))/(Amp_sf)) + (Amp_sf+min_sf)
  sat(u) : Outport
  wires:
  Manual Switch/1 -> sat(u)/1
  Saturation1/1 -> Manual Switch/2
  u/1 -> saturation function/1, apply for lower bound only/2, Mux3/1, apply for lower bound only/1, Saturation1/1
  saturation function/1 -> apply for lower bound only/3, Mux3/2
  Mux3/1 -> sat/1
  apply for lower bound only/1 -> Manual Switch/1

== system Marine_LocoMotive_UAV_est_git/UAV controller/u_r_p_Lyapunov radial position/Enabled Subsystem ==
  u : Inport
  reset : Inport  Port=2
  Enable : EnablePort
  Logical Operator : Logic  Operator=NOT  AllPortsSameDT=off  OutDataTypeStr=boolean
  Low Pass Filter5 : DiscreteTransferFcn  Numerator=Bm_reL_LPF  Denominator=Am_reL_LPF  ExternalReset=Level
      settings: InputPortMap=u0,r7
  y : Outport
  wires:
  u/1 -> Low Pass Filter5/1
  Low Pass Filter5/1 -> y/1
  Logical Operator/1 -> Low Pass Filter5/2
  reset/1 -> Logical Operator/1

== system Marine_LocoMotive_UAV_est_git/UAV controller/u_r_p_Lyapunov radial position/cond ==
  In1 : Inport
  Bias : Bias  Bias=-Lc_0
  Compare To Constant : simulink/Logic and Bit Operations/Compare To Constant  relop=<=  const=0.1  OutDataTypeStr=boolean
  Out1 : Outport
  wires:
  Bias/1 -> Compare To Constant/1
  Compare To Constant/1 -> Out1/1
  In1/1 -> Bias/1

== system Marine_LocoMotive_UAV_est_git/UAV controller/u_r_p_Lyapunov radial position/smooth lower bound ==
  u : Inport
  Manual Switch : ManualSwitch
  Mux3 : Mux  Inputs=2
  Saturation1 : Saturate  UpperLimit=inf  LowerLimit=min_sf_rp
  apply for lower bound only : Switch  Criteria=u2 > Threshold  Threshold=Amp_sf_rp+min_sf_rp
  sat : Scope
  saturation function : Fcn  Expr=Amp_sf_rp*tanh((u(1)-(Amp_sf_rp+min_sf_rp))/(Amp_sf_rp)) + (Amp_sf_rp+min_sf_rp)
  sat(u) : Outport
  wires:
  Manual Switch/1 -> sat(u)/1
  Saturation1/1 -> Manual Switch/2
  u/1 -> saturation function/1, apply for lower bound only/2, Mux3/1, apply for lower bound only/1, Saturation1/1
  saturation function/1 -> apply for lower bound only/3, Mux3/2
  Mux3/1 -> sat/1
  apply for lower bound only/1 -> Manual Switch/1

== system Marine_LocoMotive_UAV_est_git/Preprocessing Unit/T_bar /Damping coefficient estimation/Vol_im_bar to Dh_bar ==
  V : Inport
  Constant : Constant  Value=Vol_b
  Dh bar : Scope
  Product : Product
  Vol im ratio : Product  Inputs=*/
  height : Constant  Value=h_b
  D : Outport
  wires:
  V/1 -> Vol im ratio/1
  Vol im ratio/1 -> Product/2
  height/1 -> Product/1
  Product/1 -> Dh bar/1, D/1
  Constant/1 -> Vol im ratio/2

== system Marine_LocoMotive_UAV_est_git/Preprocessing Unit/T_bar /Damping coefficient estimation/advanced damping estimates ==
  Vr_bar : Inport
  Dh_bar : Inport  Port=2
  C_S : Inport  Port=3
  Abs : Abs
  Bias2 : Bias  Bias=b_11
  Constant : Constant  Value=D_x
  Constant2 : Constant  Value=0.5*rho_w
  "D11  " : Scope
  Dx : Scope
  Gain1 : Gain  Gain=2*l_b
  Manual Switch : ManualSwitch  CurrentSetting=0
  Product6 : Product  Inputs=4
  Sum5 : Sum  Inputs=|++  SaturateOnIntegerOverflow=on
  bottom plan : Constant  Value=l_b*h_b
  D11 : Outport
  wires:
  Constant2/1 -> Product6/3
  Abs/1 -> Product6/1
  Gain1/1 -> Sum5/1
  Sum5/1 -> Product6/2  "Aw"
  Dh_bar/1 -> Gain1/1
  bottom plan/1 -> Sum5/2
  C_S/1 -> Product6/4
  Vr_bar/1 -> Abs/1
  Product6/1 -> Bias2/1
  Bias2/1 -> "D11  "/1, Manual Switch/2
  Manual Switch/1 -> D11/1
  Constant/1 -> Manual Switch/1, Dx/1

== system Marine_LocoMotive_UAV_est_git/Preprocessing Unit/T_bar /Damping coefficient estimation/damping estimates ==
  V_bar : Inport
  C_S_bar : Inport  Port=2
  Abs1 : Abs
  Bias : Bias  Bias=h_b/2
  Bias2 : Bias  Bias=b_11
  Constant : Constant  Value=D_x
  Constant2 : Constant  Value=0.5*rho_w
  "D11  " : Scope
  Dh @ no tension : Constant  Value=Delta_h
  Dx : Scope
  Dx1 : Scope
  Gain1 : Gain  Gain=2*l_b
  Manual Switch : ManualSwitch  CurrentSetting=0
  Product6 : Product  Inputs=4
  Saturation : Saturate  UpperLimit=h_b  LowerLimit=0
  Sum5 : Sum  Inputs=|++  SaturateOnIntegerOverflow=on
  bottom plan : Constant  Value=l_b*h_b
  D11,0 : Outport
  wires:
  Constant/1 -> Dx/1, Manual Switch/1
  Manual Switch/1 -> D11,0/1
  Bias2/1 -> Manual Switch/2, "D11  "/1
  Product6/1 -> Bias2/1
  C_S_bar/1 -> Product6/4
  bottom plan/1 -> Sum5/2
  Dh @ no tension/1 -> Bias/1
  Sum5/1 -> Dx1/1, Product6/2  "Aw"
  Gain1/1 -> Sum5/1
  V_bar/1 -> Abs1/1
  Constant2/1 -> Product6/3
  Abs1/1 -> Product6/1
  Bias/1 -> Saturation/1
  Saturation/1 -> Gain1/1

== system Marine_LocoMotive_UAV_est_git/Preprocessing Unit/T_bar /Damping coefficient estimation/mean skin friction coefficient  ==
  V : Inport
  Abs1 : Abs
  C_S Lewis1988 : Fcn  Expr=0.075/(log10(u(1))-2)^2
  Re Reynolds number : Gain  Gain=l_b/nu_w
  Saturation1 : Saturate  UpperLimit=inf  LowerLimit=0.5*10^5
  C_S : Outport
  wires:
  Re Reynolds number/1 -> Saturation1/1
  Abs1/1 -> Re Reynolds number/1
  Saturation1/1 -> C_S Lewis1988/1
  V/1 -> Abs1/1
  C_S Lewis1988/1 -> C_S/1

== system Marine_LocoMotive_UAV_est_git/Quadrotor+buoy/3-DOF equations of motion Earth frame/D_123/Water Daming ==
  theta_b : Inport
  eta_dot_tilde : Inport  Port=2
  dh : Inport  Port=3
  Abs : Abs
  Abs3 : Abs
  Add1 : Sum
  Add2 : Sum
  Add3 : Sum  Inputs=+-
  Bias : Bias  Bias=h_b/2
  Bias2 : Bias  Bias=b_11
  Bias3 : Bias  Bias=b_33
  C_S : Fcn  Expr=0.075/(log10(u(1))-2)^2
  C_S Lewis1988 : Fcn  Expr=0.075/(log10(u(1))-2)^2
  Constant1 : Constant  Value=0.5*rho_w
  Constant13 : Constant  Value=2
  Constant3 : Constant  Value=C_S
  Gain : Gain  Gain=2
  Gain1 : Gain  Gain=2*l_b
  Manual Switch : ManualSwitch  CurrentSetting=0
  Math Function : Math  Operator=transpose  SaturateOnIntegerOverflow=on
  Product{,6..8} (4 alike) : Product  Inputs=3
  Product1 : Product  Inputs=4
  Product9 : Product  Inputs=**/
  Re Reynolds number : Gain  Gain=l_b/nu_w
  Re_Vbx : Selector  InputPortWidth=2  IndexOptions=Index vector (dialog)  Indices=1  OutputSizes=1
  Re_Vbz : Selector  InputPortWidth=2  IndexOptions=Index vector (dialog)  Indices=2  OutputSizes=1
  Saturation : Saturate  UpperLimit=h_b  LowerLimit=0
  Saturation1 : Saturate  UpperLimit=inf  LowerLimit=0.5*10^5
  Scope2 : Scope
  Scope5 : Scope
  Scope6 : Scope
  Selector : Selector  InputPortWidth=3  IndexOptions=Index vector (dialog)  Indices=[1 2]  OutputSizes=1
  Signal Specification : SignalSpecification  Dimensions=1
  Signal Specification1 : SignalSpecification  Dimensions=1
  Sum5 : Sum  Inputs=|++  SaturateOnIntegerOverflow=on
  Trigonometric Function1 : Trigonometry  Operator=sincos
  Trigonometric Function2 : Trigonometry  Operator=sincos
  Trigonometric Function3 : Trigonometry
  Vector Concatenate : Concatenate
  bottom plan : Constant  Value=l_b*h_b
  rotation matrix R body to earth : Subsystem
  "tilde{nu}_12" : Product  Multiplication=Matrix(*)
  x : Selector  InputPortWidth=2  IndexOptions=Index vector (dialog)  Indices=1  OutputSizes=1
  z : Selector  InputPortWidth=2  IndexOptions=Index vector (dialog)  Indices=1  OutputSizes=1
  D11_I : Outport
  D22_I : Outport  Port=2
  D12_I : Outport  Port=3
  wires:
  Constant13/1 -> Product9/3
  Product7/1 -> Add2/1
  Add3/1 -> Product9/2
  Bias2/1 -> Add3/2, Product7/1, Product6/3
  Bias3/1 -> Add3/1, Product8/3, Product/1
  Product/1 -> Add1/1
  Product6/1 -> Add1/2
  Product8/1 -> Add2/2
  Trigonometric Function1/2 -> Product6/2, Product6/1
  Trigonometric Function2/1 -> Product7/3, Product7/2
  Trigonometric Function2/2 -> Product8/1, Product8/2
  z/1 -> Bias3/1
  Trigonometric Function3/1 -> Product9/1
  Trigonometric Function1/1 -> Product/2, Product/3
  Product9/1 -> D12_I/1
  Gain/1 -> Trigonometric Function3/1
  theta_b/1 -> rotation matrix R body to earth/1(angle (rad)), Gain/1, Trigonometric Function2/1, Trigonometric Function1/1
  rotation matrix R body to earth/1(R) -> Math Function/1
  eta_dot_tilde/1 -> Selector/1
  Math Function/1 -> "tilde{nu}_12"/1
  dh/1 -> Bias/1
  Gain1/1 -> Sum5/1
  bottom plan/1 -> Sum5/2
  Sum5/1 -> Product1/2  "Aw"
  Constant1/1 -> Product1/3
  Manual Switch/1 -> Product1/4  "C_S"
  x/1 -> Bias2/1
  "tilde{nu}_12"/1 -> Abs3/1
  Signal Specification/1 -> D11_I/1
  Add1/1 -> Signal Specification/1
  Add2/1 -> Signal Specification1/1
  Signal Specification1/1 -> D22_I/1
  Product1/1 -> z/1, x/1
  Re Reynolds number/1 -> Scope6/1, Saturation1/1
  Constant3/1 -> Manual Switch/1
  C_S Lewis1988/1 -> Vector Concatenate/2
  C_S/1 -> Vector Concatenate/1
  Bias/1 -> Scope5/1, Saturation/1
  Saturation/1 -> Gain1/1
  Re_Vbx/1 -> C_S/1
  Re_Vbz/1 -> C_S Lewis1988/1
  Saturation1/1 -> Re_Vbz/1, Re_Vbx/1
  Selector/1 -> "tilde{nu}_12"/2, Abs/1  "don't put the |.| here!!"
  Abs3/1 -> Product1/1  "nu_tilde_bar"
  Abs/1 -> Re Reynolds number/1
  Vector Concatenate/1 -> Scope2/1, Manual Switch/2

== system Marine_LocoMotive_UAV_est_git/Quadrotor+buoy/3-DOF equations of motion Earth frame/D_123/Water Daming1 ==
  theta : Inport
  Add1 : Sum
  Add2 : Sum
  Add3 : Sum  Inputs=+-
  Constant10 : Constant  Value=D_z
  Constant11 : Constant  Value=D_x
  Constant12 : Constant  Value=D_z
  Constant13 : Constant  Value=2
  Constant7 : Constant  Value=D_x
  Constant8 : Constant  Value=D_z
  Constant9 : Constant  Value=D_x
  Gain : Gain  Gain=2
  Product{,6..8} (4 alike) : Product  Inputs=3
  Product9 : Product  Inputs=**/
  Trigonometric Function1 : Trigonometry  Operator=sincos
  Trigonometric Function2 : Trigonometry  Operator=sincos
  Trigonometric Function3 : Trigonometry
  D11_I : Outport
  D22_I : Outport  Port=2
  D12_I : Outport  Port=3
  wires:
  Gain/1 -> Trigonometric Function3/1
  Add1/1 -> D11_I/1
  Product9/1 -> D12_I/1
  theta/1 -> Trigonometric Function1/1, Trigonometric Function2/1, Gain/1
  Trigonometric Function1/1 -> Product/3, Product/2
  Trigonometric Function3/1 -> Product9/1
  Constant8/1 -> Product/1
  Trigonometric Function2/2 -> Product8/2, Product8/1
  Trigonometric Function2/1 -> Product7/2, Product7/3
  Trigonometric Function1/2 -> Product6/1, Product6/2
  Product8/1 -> Add2/2
  Add2/1 -> D22_I/1
  Product6/1 -> Add1/2
  Product/1 -> Add1/1
  Constant10/1 -> Product8/3
  Constant12/1 -> Add3/1
  Constant7/1 -> Product6/3
  Constant11/1 -> Add3/2
  Add3/1 -> Product9/2
  Product7/1 -> Add2/1
  Constant13/1 -> Product9/3
  Constant9/1 -> Product7/1

== system Marine_LocoMotive_UAV_est_git/Quadrotor+buoy/3-DOF equations of motion Earth frame/M_12/added mass ==
  theta : Inport
  Add1 : Sum
  Add2 : Sum
  Add3 : Sum  Inputs=+-
  Constant13 : Constant  Value=2
  Gain : Gain  Gain=2
  M11 : Constant  Value=m_b+a_ii(1)
  "M11 " : Constant  Value=m_b+a_ii(1)
  M11 1 : Constant  Value=m_b+a_ii(1)
  "M22 " : Constant  Value=m_b+a_ii(2)
  M22 1 : Constant  Value=m_b+a_ii(2)
  M_22 : Constant  Value=m_b+a_ii(2)
  Product{,6..8} (4 alike) : Product  Inputs=3
  Product9 : Product  Inputs=**/
  Trigonometric Function1 : Trigonometry  Operator=sincos
  Trigonometric Function2 : Trigonometry  Operator=sincos
  Trigonometric Function3 : Trigonometry
  M11_I : Outport
  M22_I : Outport  Port=2
  M12_I : Outport  Port=3
  wires:
  Gain/1 -> Trigonometric Function3/1
  "M11 "/1 -> Product7/1
  Constant13/1 -> Product9/3
  Product7/1 -> Add2/1
  Add3/1 -> Product9/2
  M11 1/1 -> Add3/2
  M11/1 -> Product6/3
  M22 1/1 -> Add3/1
  "M22 "/1 -> Product8/3
  Product/1 -> Add1/1
  Product6/1 -> Add1/2
  Add2/1 -> M22_I/1
  Product8/1 -> Add2/2
  Trigonometric Function1/2 -> Product6/2, Product6/1
  Trigonometric Function2/1 -> Product7/3, Product7/2
  Trigonometric Function2/2 -> Product8/1, Product8/2
  M_22/1 -> Product/1
  Trigonometric Function3/1 -> Product9/1
  Trigonometric Function1/1 -> Product/2, Product/3
  theta/1 -> Gain/1, Trigonometric Function2/1, Trigonometric Function1/1
  Product9/1 -> M12_I/1
  Add1/1 -> M11_I/1

== system Marine_LocoMotive_UAV_est_git/Quadrotor+buoy/3-DOF equations of motion Earth frame/M_123/buoy inertia ==
  theta : Inport
  Add1 : Sum
  Add2 : Sum
  Add3 : Sum  Inputs=+-
  Constant13 : Constant  Value=2
  Gain : Gain  Gain=2
  M11 : Constant  Value=m_b+a_ii(1)
  "M11 " : Constant  Value=m_b+a_ii(1)
  M11 1 : Constant  Value=m_b+a_ii(1)
  "M22 " : Constant  Value=m_b+a_ii(2)
  M22 1 : Constant  Value=m_b+a_ii(2)
  M_22 : Constant  Value=m_b+a_ii(2)
  Product{,6..8} (4 alike) : Product  Inputs=3
  Product9 : Product  Inputs=**/
  Trigonometric Function1 : Trigonometry  Operator=sincos
  Trigonometric Function2 : Trigonometry  Operator=sincos
  Trigonometric Function3 : Trigonometry
  M11_I : Outport
  M22_I : Outport  Port=2
  M12_I : Outport  Port=3
  wires:
  Add1/1 -> M11_I/1
  Product9/1 -> M12_I/1
  theta/1 -> Trigonometric Function1/1, Trigonometric Function2/1, Gain/1
  Trigonometric Function1/1 -> Product/3, Product/2
  Trigonometric Function3/1 -> Product9/1
  M_22/1 -> Product/1
  Trigonometric Function2/2 -> Product8/2, Product8/1
  Trigonometric Function2/1 -> Product7/2, Product7/3
  Trigonometric Function1/2 -> Product6/1, Product6/2
  Product8/1 -> Add2/2
  Add2/1 -> M22_I/1
  Product6/1 -> Add1/2
  Product/1 -> Add1/1
  "M22 "/1 -> Product8/3
  M22 1/1 -> Add3/1
  M11/1 -> Product6/3
  M11 1/1 -> Add3/2
  Add3/1 -> Product9/2
  Product7/1 -> Add2/1
  Constant13/1 -> Product9/3
  "M11 "/1 -> Product7/1
  Gain/1 -> Trigonometric Function3/1

== system Marine_LocoMotive_UAV_est_git/Quadrotor+buoy/3-DOF equations of motion Earth frame/Quadrotor Dynamics Outer-Loop/Gu ==
  coupled : Inport
  Constant3 : Constant  Value=0
  Constant4 : Constant  Value=m_u
  Gain1 : Gain  Gain=g
  Product : Product
  Vector Concatenate : Concatenate
  G : Outport
  wires:
  Product/1 -> Gain1/1
  Constant4/1 -> Product/2  "u2"
  coupled/1 -> Product/1
  Vector Concatenate/1 -> G/1
  Constant3/1 -> Vector Concatenate/1  "u1"
  Gain1/1 -> Vector Concatenate/2  "u2"
